simulink model "UDSservices"  (R2024a)
settings: Solver=VariableStepAuto  StartTime=0.0  StopTime=10.0  RelTol=1e-3
undefined symbols (not defined in the file or in its folder): canChannel
libraries: canlib x7, simulink x6, canmsglib x5
settings Model: DataDictionary=BMS_System_dict1.sldd  Creator=hirah  LastModifiedBy=hirah

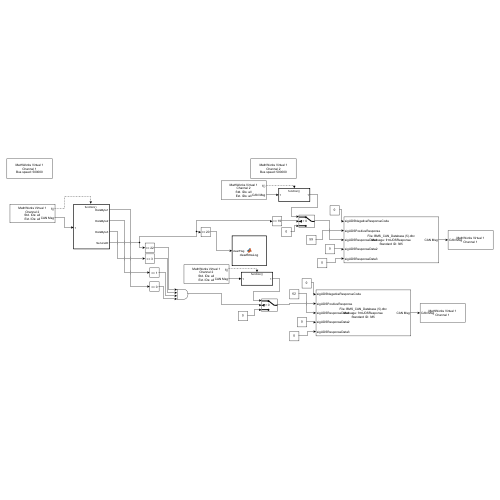
[thumbnail: Simulink's stored preview of the top-level diagram]
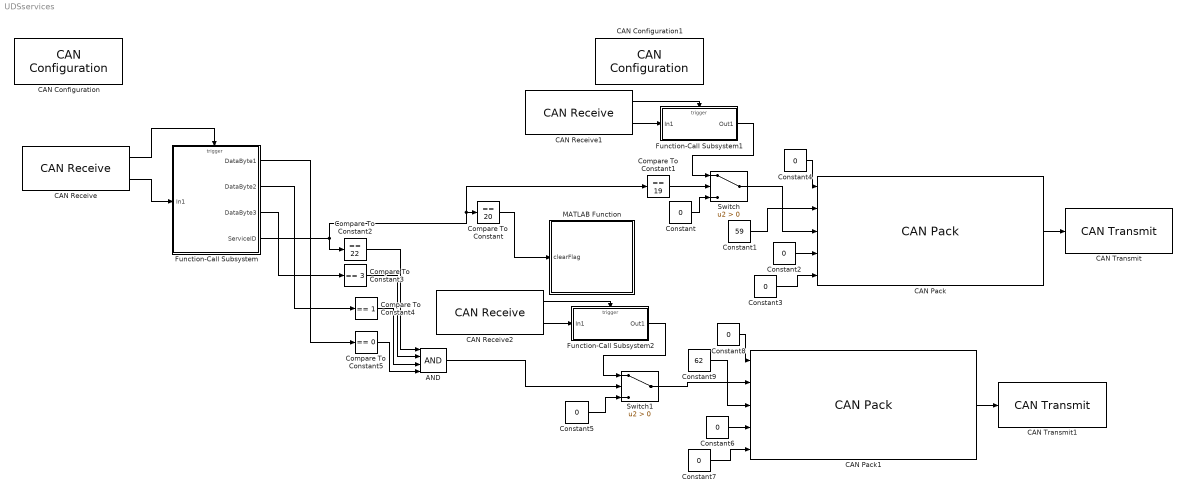
== system UDSservices ==
  AND : Logic  Inputs=4  IconShape=distinctive  AllPortsSameDT=off  OutDataTypeStr=boolean
  CAN Configuration : canlib/CAN Configuration  BlockHandle=570.0001  Device=MathWorks Virtual 1 (Channel 1)  DeviceMenu=MathWorks Virtual 1 (Channel 1)  ObjConstructor=canChannel('MathWorks', 'Virtual 1', 1)  BusSpeed=500000  EnableBitParameters=off  AckMode=Normal
  CAN Configuration1 : canlib/CAN Configuration  BlockHandle=570.0001  Device=MathWorks Virtual 1 (Channel 2)  DeviceMenu=MathWorks Virtual 1 (Channel 2)  ObjConstructor=canChannel('MathWorks', 'Virtual 1', 2)  BusSpeed=500000  EnableBitParameters=off  AckMode=Normal
  CAN Pack : canmsglib/CAN Pack  CANdbFile=C:\Users\hirah\Downloads\BMS_CAN_Database (5).dbc  MsgList=frmUDSResponse  MsgName=frmUDSResponse  MsgIDType=Standard (11-bit identifier)  MsgIdentifier=385  MsgLength=8  Remote=off  ApplyMinMax=off  BusOutput=off  SignalInfo={ 'sigUDSNegativeResponseCode', '32', '8', 'LE', 'unsigned', 'Standard', '0', '1', '0', '0', '255'; 'sigUDSPositiveResponse', '0', '8', 'LE', 'unsigned', 'Standard', '0', '1', '0', '0', '255'; 'sigUDSResponseData1', '8', '8', 'LE', 'unsigned', 'Standard', '0', '1', '0', '0', '255'; 'sigUDSResponseData2', '16', '8', 'LE', 'unsigned', 'Standard', '0', '1', '0', '0', '255'; 'sigUDSResponseData3', '24', '8', 'LE', 'unsigned', 'Standard', '0', '1', '0', '0', '255' }
      settings: LibrarySourceBlock=canlib/CAN Pack  DataFormat=CANdb specified signals
  CAN Pack1 : canmsglib/CAN Pack  CANdbFile=C:\Users\hirah\Downloads\BMS_CAN_Database (5).dbc  MsgList=frmUDSResponse  MsgName=frmUDSResponse  MsgIDType=Standard (11-bit identifier)  MsgIdentifier=385  MsgLength=8  Remote=off  ApplyMinMax=off  BusOutput=off  SignalInfo={'sigUDSNegativeResponseCode','32','8','LE','unsigned','Standard','0','1','0','0','255';'sigUDSPositiveResponse','0','8','LE','unsigned','Standard','0','1','0','0','255';'sigUDSResponseData1','8','8','LE','unsigned','Standard','0','1','0','0','255';'sigUDSResponseData2','16','8','LE','unsigned','Standard','0','1','0','0','255';'sigUDSResponseData3','24','8','LE','unsigned','Standard','0','1','0','0','255'}
      settings: LibrarySourceBlock=canlib/CAN Pack  DataFormat=CANdb specified signals
  CAN Receive : canlib/CAN Receive  BlockHandle=729.0002  Device=MathWorks Virtual 1 (Channel 2)  DeviceMenu=MathWorks Virtual 1 (Channel 2)  ObjConstructor=canChannel('MathWorks', 'Virtual 1', 2)  EnableStandardIDsFilter=off  StdIDsCombo=Allow all  StandardIDs=261  EnableExtendedIDsFilter=off  ExtIDsCombo=Allow all  ExtendedIDs=0  SampleTime=0.01  MsgsPerTimestep=all  InternalFilterUpdateStatus=on  BusOutput=off
  CAN Receive1 : canlib/CAN Receive  BlockHandle=729.0002  Device=MathWorks Virtual 1 (Channel 2)  DeviceMenu=MathWorks Virtual 1 (Channel 2)  ObjConstructor=canChannel('MathWorks', 'Virtual 1', 2)  EnableStandardIDsFilter=off  StdIDsCombo=Allow all  StandardIDs=261  EnableExtendedIDsFilter=off  ExtIDsCombo=Allow all  ExtendedIDs=0  SampleTime=0.01  MsgsPerTimestep=all  InternalFilterUpdateStatus=on  BusOutput=off
  CAN Receive2 : canlib/CAN Receive  BlockHandle=729.0002  Device=MathWorks Virtual 1 (Channel 2)  DeviceMenu=MathWorks Virtual 1 (Channel 2)  ObjConstructor=canChannel('MathWorks', 'Virtual 1', 2)  EnableStandardIDsFilter=off  StdIDsCombo=Allow all  StandardIDs=261  EnableExtendedIDsFilter=off  ExtIDsCombo=Allow all  ExtendedIDs=0  SampleTime=0.01  MsgsPerTimestep=all  InternalFilterUpdateStatus=on  BusOutput=off
  CAN Transmit : canlib/CAN Transmit  BlockHandle=714.0001  Device=MathWorks Virtual 1 (Channel 1)  DeviceMenu=MathWorks Virtual 1 (Channel 1)  ObjConstructor=canChannel('MathWorks', 'Virtual 1', 1)  EnableEventTransmit=off  EnablePeriodicTransmit=off  MessagePeriod=1.000
  CAN Transmit1 : canlib/CAN Transmit  BlockHandle=714.0001  Device=MathWorks Virtual 1 (Channel 1)  DeviceMenu=MathWorks Virtual 1 (Channel 1)  ObjConstructor=canChannel('MathWorks', 'Virtual 1', 1)  EnableEventTransmit=off  EnablePeriodicTransmit=off  MessagePeriod=1.000
  Compare To Constant : simulink/Logic and Bit Operations/Compare To Constant  relop===  const=20  OutDataTypeStr=boolean
  Compare To Constant1 : simulink/Logic and Bit Operations/Compare To Constant  relop===  const=19  OutDataTypeStr=boolean
  Compare To Constant2 : simulink/Logic and Bit Operations/Compare To Constant  relop===  const=22  OutDataTypeStr=boolean
  Compare To Constant3 : simulink/Logic and Bit Operations/Compare To Constant  relop===  const=3  OutDataTypeStr=boolean
  Compare To Constant4 : simulink/Logic and Bit Operations/Compare To Constant  relop===  const=1  OutDataTypeStr=boolean
  Compare To Constant5 : simulink/Logic and Bit Operations/Compare To Constant  relop===  const=0  OutDataTypeStr=boolean
  Constant{,2..8} (8 alike) : Constant  Value=0
  Constant1 : Constant  Value=59
  Constant9 : Constant  Value=62
  Function-Call Subsystem : Subsystem  TreatAsAtomicUnit=on
  Function-Call Subsystem1 : Subsystem  TreatAsAtomicUnit=on
  Function-Call Subsystem2 : Subsystem  TreatAsAtomicUnit=on
  MATLAB Function : MATLAB Function  TreatAsAtomicUnit=on
  Switch : Switch  Criteria=u2 > Threshold  SaturateOnIntegerOverflow=off  InputSameDT=off
  Switch1 : Switch  Criteria=u2 > Threshold  SaturateOnIntegerOverflow=off  InputSameDT=off
  wires:
  CAN Receive/2 -> Function-Call Subsystem/1(In1)
  CAN Receive/1 -> Function-Call Subsystem/Trigger
  Function-Call Subsystem/4(ServiceID) -> Compare To Constant1/1, Compare To Constant/1, Compare To Constant2/1
  Compare To Constant/1 -> MATLAB Function/1(clearFlag)
  Compare To Constant1/1 -> Switch/2
  Constant/1 -> Switch/3
  CAN Receive1/2 -> Function-Call Subsystem1/1(In1)
  CAN Receive1/1 -> Function-Call Subsystem1/Trigger
  Function-Call Subsystem1/1(Out1) -> Switch/1
  CAN Pack/1 -> CAN Transmit/1
  Switch/1 -> CAN Pack/3
  Constant1/1 -> CAN Pack/2
  Constant2/1 -> CAN Pack/4
  Constant3/1 -> CAN Pack/5
  Constant4/1 -> CAN Pack/1
  Function-Call Subsystem/3(DataByte3) -> Compare To Constant3/1
  Function-Call Subsystem/2(DataByte2) -> Compare To Constant4/1
  Function-Call Subsystem/1(DataByte1) -> Compare To Constant5/1
  Compare To Constant2/1 -> AND/1
  Compare To Constant3/1 -> AND/2
  Compare To Constant4/1 -> AND/3
  Compare To Constant5/1 -> AND/4
  Function-Call Subsystem2/1(Out1) -> Switch1/1
  CAN Receive2/2 -> Function-Call Subsystem2/1(In1)
  CAN Receive2/1 -> Function-Call Subsystem2/Trigger
  AND/1 -> Switch1/2
  Constant5/1 -> Switch1/3
  Switch1/1 -> CAN Pack1/2
  Constant6/1 -> CAN Pack1/4
  Constant7/1 -> CAN Pack1/5
  Constant8/1 -> CAN Pack1/1
  CAN Pack1/1 -> CAN Transmit1/1
  Constant9/1 -> CAN Pack1/3

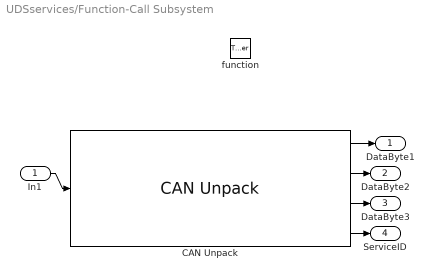
== system UDSservices/Function-Call Subsystem ==
  In1 : Inport
  function : TriggerPort  TriggerType=function-call  VariantControl=(inherit)
  CAN Unpack : canmsglib/CAN Unpack  CANdbFile=C:\Users\hirah\Downloads\BMS_CAN_Database (5).dbc  MsgList=frmUDSRequest  MsgName=frmUDSRequest  MsgIDType=Standard (11-bit identifier)  MsgIdentifier=384  MsgLength=8  SignalInfo={ 'sigUDSDataByte1', '16', '8', 'LE', 'unsigned', 'Standard', '0', '1', '0', '0', '255'; 'sigUDSDataByte2', '24', '8', 'LE', 'unsigned', 'Standard', '0', '1', '0', '0', '255'; 'sigUDSDataByte3', '32', '8', 'LE', 'unsigned', 'Standard', '0', '1', '0', '0', '255'; 'sigUDSServiceID', '0', '8', 'LE', 'unsigned', 'Standard', '0', '1', '0', '0', '255' }  IDPort=off  TimestampPort=off  ErrorPort=off  RemotePort=off  LengthPort=off  StatusPort=off  ApplyMinMax=off
  DataByte1 : Outport
  DataByte2 : Outport  Port=2
  DataByte3 : Outport  Port=3
  ServiceID : Outport  Port=4
  wires:
  In1/1 -> CAN Unpack/1
  CAN Unpack/1 -> DataByte1/1
  CAN Unpack/2 -> DataByte2/1
  CAN Unpack/3 -> DataByte3/1
  CAN Unpack/4 -> ServiceID/1

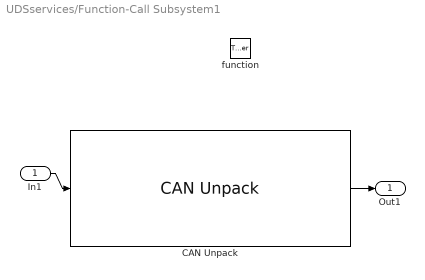
== system UDSservices/Function-Call Subsystem1 ==
  In1 : Inport
  function : TriggerPort  TriggerType=function-call  VariantControl=(inherit)
  CAN Unpack : canmsglib/CAN Unpack  CANdbFile=C:\Users\hirah\Downloads\BMS_CAN_Database (5).dbc  MsgList=frmDiagnosticDTC  MsgName=frmDiagnosticDTC  MsgIDType=Standard (11-bit identifier)  MsgIdentifier=264  MsgLength=3  SignalInfo={ 'sigDTCCode1', '0', '16', 'LE', 'unsigned', 'Standard', '0', '1', '0', '0', '65535' }  IDPort=off  TimestampPort=off  ErrorPort=off  RemotePort=off  LengthPort=off  StatusPort=off  ApplyMinMax=off
  Out1 : Outport
  wires:
  In1/1 -> CAN Unpack/1
  CAN Unpack/1 -> Out1/1

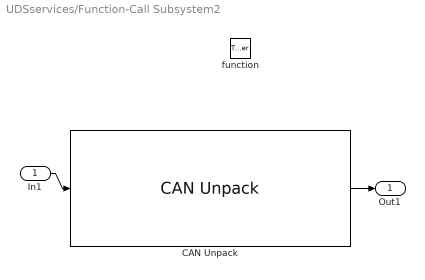
== system UDSservices/Function-Call Subsystem2 ==
  In1 : Inport
  function : TriggerPort  TriggerType=function-call  VariantControl=(inherit)
  CAN Unpack : canmsglib/CAN Unpack  CANdbFile=C:\Users\hirah\Downloads\BMS_CAN_Database (5).dbc  MsgList=frmBMStoVCU  MsgName=frmBMStoVCU  MsgIDType=Standard (11-bit identifier)  MsgIdentifier=321  MsgLength=2  SignalInfo={ 'sigBMSOperatingMode', '0', '8', 'LE', 'unsigned', 'Standard', '0', '1', '0', '0', '5' }  IDPort=off  TimestampPort=off  ErrorPort=off  RemotePort=off  LengthPort=off  StatusPort=off  ApplyMinMax=off
  Out1 : Outport
  wires:
  In1/1 -> CAN Unpack/1
  CAN Unpack/1 -> Out1/1

== matlab function UDSservices/MATLAB Function ==
  data: clearFlag input
function clearBmsLog(clearFlag)
% clearBmsLog  Clears (truncates) bms_log.csv if clearFlag is true.
%
% Usage:
%   clearBmsLog(true)   % clears the file
%   clearBmsLog(false)  % does nothing

    if nargin ~= 1
        error('1 input required: clearFlag');
    end

    filename = 'bms_log.csv';

    if ~islogical(clearFlag) && ~isnumeric(clearFlag)
        error('clearFlag must be logical or numeric.');
    end

    if logical(clearFlag)
        if isfile(filename)
            fid = fopen(filename, 'w');   % 'w' truncates file
            if fid == -1
                error('Failed to open %s for clearing.', filename);
            end
            fclose(fid);
        end
    end
end
